simulink model "linear_extended"  (R2017b)
settings: Solver=VariableStepAuto  StartTime=0.0  StopTime=10.0  RelTol=1e-3
undefined symbols (not defined in the file): pars, system
settings Model: Creator=Twan  LastModifiedBy=Twan

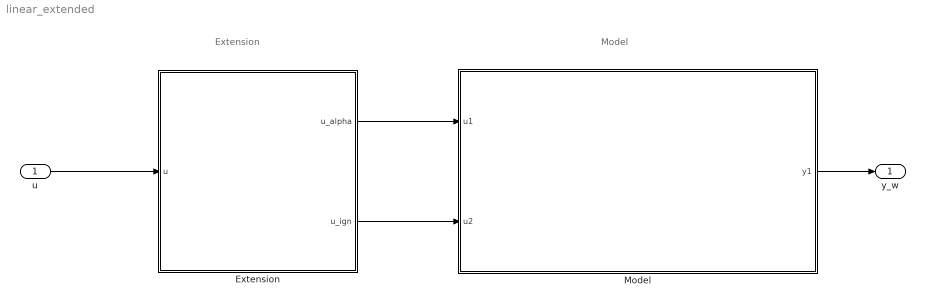
== system linear_extended ==
  note: Extension
  note: Model
  u : Inport
  "Extension " : Subsystem
  Model : Subsystem
  "y_w " : Outport
  wires:
  Model/1(y1) -> "y_w "/1
  "Extension "/1(u_alpha) -> Model/1(u1)
  "Extension "/2(u_ign) -> Model/2(u2)
  u/1 -> "Extension "/1(u)

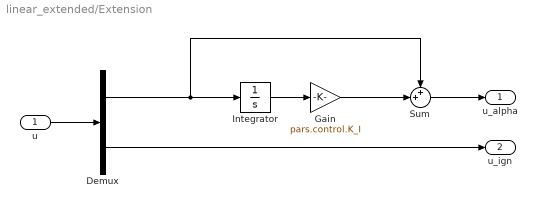
== system linear_extended/Extension  ==
  u : Inport
  Demux : Demux  Outputs=2
  Gain : Gain  Gain=pars.control.K_I
  Integrator : Integrator
  Sum : Sum  Inputs=++|
  u_alpha : Outport
  u_ign : Outport  Port=2
  wires:
  u/1 -> Demux/1
  Demux/1 -> Sum/1, Integrator/1
  Integrator/1 -> Gain/1
  Sum/1 -> u_alpha/1
  Demux/2 -> u_ign/1
  Gain/1 -> Sum/2

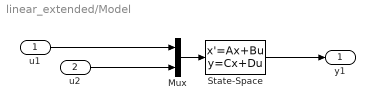
== system linear_extended/Model ==
  u1 : Inport
  u2 : Inport  Port=2
  Mux : Mux  Inputs=2
  State-Space : StateSpace  A=system.ss.lin.A  B=system.ss.lin.B  C=system.ss.lin.C  D=system.ss.lin.D  InitialCondition=[1]
  y1 : Outport
  wires:
  Mux/1 -> State-Space/1
  u1/1 -> Mux/1
  u2/1 -> Mux/2
  State-Space/1 -> y1/1
